simulink model "TP"  (R2021a)
settings: Solver=VariableStepAuto  StartTime=0.0  StopTime=T  MaxStep=0.01  RelTol=1e-6
undefined symbols (not defined in the file): A, A0, A0_, algorithmSelect, b, C, e1, e2, gamma, theta
settings Model: Creator=X-X  LastModifiedBy=fussybaby
settings SolverCC: AlgebraicLoopSolver=TrustRegion
settings DebuggingCC: SFMachineParentedDataDiag=warning

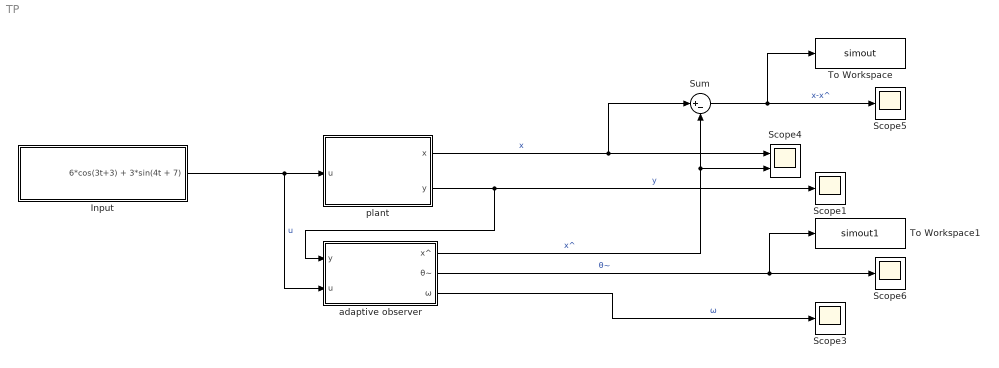
== system TP ==
  Input : Subsystem
  Scope{1,3,5..6} (4 alike) : Scope
  Scope4 : Scope  NumInputPorts=2
  Sum : Sum  Inputs=|+-
  To Workspace : ToWorkspace  VariableName=simout  SaveFormat=Timeseries  SampleTime=-1
  To Workspace1 : ToWorkspace  VariableName=simout1  SaveFormat=Timeseries  SampleTime=-1
  adaptive observer : Subsystem
  plant : Subsystem
  wires:
  plant/2(y) -> Scope1/1, adaptive observer/1(y)  "y"
  Input/1(6*cos(3t+3) + 3*sin(4t + 7)) -> plant/1(u), adaptive observer/2(u)  "u"
  plant/1(x) -> Scope4/1, Sum/1  "x"
  adaptive observer/1(x^) -> Scope4/2, Sum/2  "x^"
  adaptive observer/2(θ~) -> To Workspace1/1, Scope6/1  "θ~"
  adaptive observer/3(ω) -> Scope3/1  "ω"
  Sum/1 -> To Workspace/1, Scope5/1  "x-x^"

== system TP/Input ==
  Sine Wave : Sin  Amplitude=-6  Frequency=3  Phase=3-pi/2  SampleTime=0
  Sine Wave1 : Sin  Amplitude=3  Frequency=4  Phase=7  SampleTime=0
  Sum : Sum  Inputs=|++
  6*cos(3t+3) + 3*sin(4t + 7) : Outport
  wires:
  Sine Wave1/1 -> Sum/2  "3*sin(4t + 7)"
  Sum/1 -> 6*cos(3t+3) + 3*sin(4t + 7)/1
  Sine Wave/1 -> Sum/1  "6*cos(3t+3)"

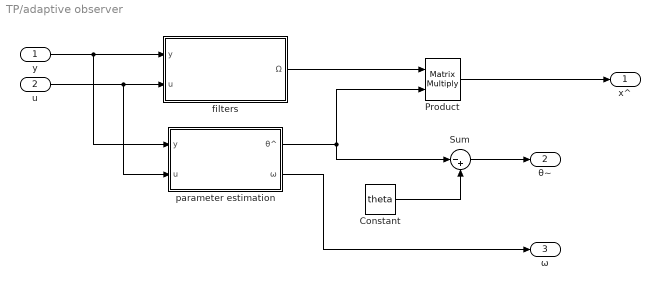
== system TP/adaptive observer ==
  y : Inport
  u : Inport  Port=2
  Constant : Constant  Value=theta
  Product : Product  Multiplication=Matrix(*)
  Sum : Sum  Inputs=|-+
  "filters " : Subsystem
  "parameter estimation " : Subsystem
  x^ : Outport
  θ~ : Outport  Port=2
  ω : Outport  Port=3
  wires:
  Product/1 -> x^/1
  y/1 -> "parameter estimation "/1(y), "filters "/1(y)
  u/1 -> "parameter estimation "/2(u), "filters "/2(u)
  "filters "/1(Ω) -> Product/1
  Constant/1 -> Sum/2
  Sum/1 -> θ~/1
  "parameter estimation "/1(θ^) -> Sum/1, Product/2
  "parameter estimation "/2(ω) -> ω/1

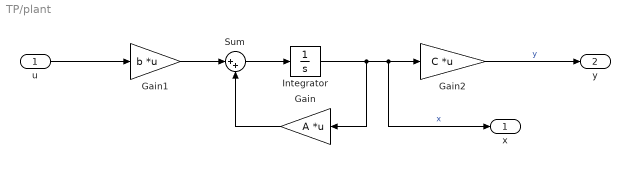
== system TP/plant ==
  u : Inport
  Gain : Gain  Gain=A  Multiplication=Matrix(K*u) (u vector)
  Gain1 : Gain  Gain=b  Multiplication=Matrix(K*u) (u vector)
  Gain2 : Gain  Gain=C  Multiplication=Matrix(K*u) (u vector)
  Integrator : Integrator  InitialCondition=[1; 0]
  Sum : Sum  Inputs=|++
  x : Outport
  y : Outport  Port=2
  wires:
  Integrator/1 -> x/1, Gain2/1, Gain/1  "x"
  Gain1/1 -> Sum/1
  Gain/1 -> Sum/2
  Sum/1 -> Integrator/1
  u/1 -> Gain1/1
  Gain2/1 -> y/1  "y"

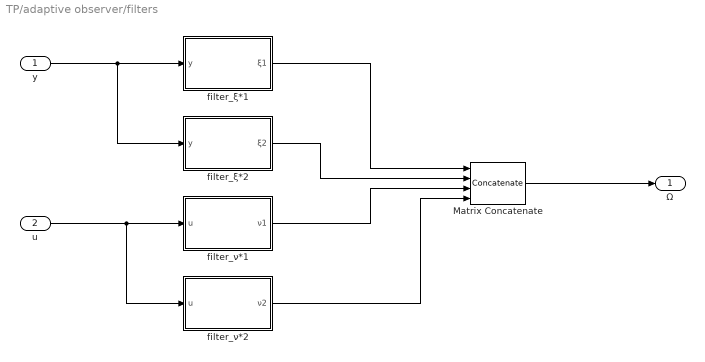
== system TP/adaptive observer/filters  ==
  y : Inport
  u : Inport  Port=2
  Matrix Concatenate : Concatenate  NumInputs=4  Mode=Multidimensional array  ConcatenateDimension=2
  filter_ν*1 : Subsystem
  filter_ν*2 : Subsystem
  filter_ξ*1 : Subsystem
  filter_ξ*2 : Subsystem
  Ω : Outport
  wires:
  y/1 -> filter_ξ*2/1(y), filter_ξ*1/1(y)
  u/1 -> filter_ν*2/1(u), filter_ν*1/1(u)
  filter_ξ*1/1(ξ1) -> Matrix Concatenate/1
  filter_ξ*2/1(ξ2) -> Matrix Concatenate/2
  filter_ν*1/1(ν1) -> Matrix Concatenate/3
  filter_ν*2/1(ν2) -> Matrix Concatenate/4
  Matrix Concatenate/1 -> Ω/1

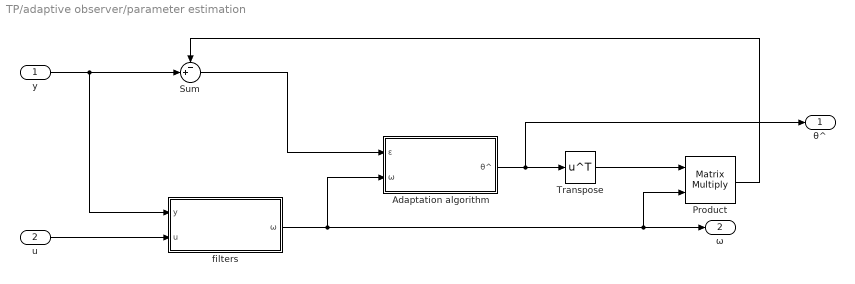
== system TP/adaptive observer/parameter estimation  ==
  y : Inport
  u : Inport  Port=2
  Adaptation algorithm : Subsystem
  Product : Product  Multiplication=Matrix(*)
  Sum : Sum  Inputs=-+|
  Transpose : Math  Operator=transpose  SaturateOnIntegerOverflow=on
  filters : Subsystem
  θ^ : Outport
  ω : Outport  Port=2
  wires:
  u/1 -> filters/2(u)
  filters/1(ω) -> Adaptation algorithm/2(ω), ω/1, Product/2
  Adaptation algorithm/1(θ^) -> θ^/1, Transpose/1
  Transpose/1 -> Product/1
  Product/1 -> Sum/1
  y/1 -> Sum/2, filters/1(y)
  Sum/1 -> Adaptation algorithm/1(ε)

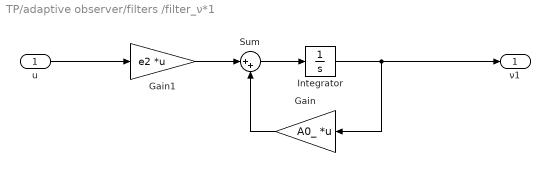
== system TP/adaptive observer/filters /filter_ν*1 ==
  u : Inport
  Gain : Gain  Gain=A0_  Multiplication=Matrix(K*u) (u vector)
  Gain1 : Gain  Gain=e2  Multiplication=Matrix(K*u) (u vector)
  Integrator : Integrator  InitialCondition=[0; 0]
  Sum : Sum  Inputs=|++
  ν1 : Outport
  wires:
  u/1 -> Gain1/1
  Gain/1 -> Sum/2
  Integrator/1 -> ν1/1, Gain/1
  Gain1/1 -> Sum/1
  Sum/1 -> Integrator/1

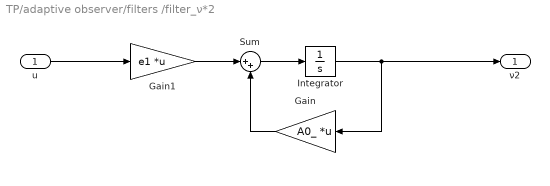
== system TP/adaptive observer/filters /filter_ν*2 ==
  u : Inport
  Gain : Gain  Gain=A0_  Multiplication=Matrix(K*u) (u vector)
  Gain1 : Gain  Gain=e1  Multiplication=Matrix(K*u) (u vector)
  Integrator : Integrator  InitialCondition=[0; 0]
  Sum : Sum  Inputs=|++
  ν2 : Outport
  wires:
  u/1 -> Gain1/1
  Gain/1 -> Sum/2
  Integrator/1 -> ν2/1, Gain/1
  Gain1/1 -> Sum/1
  Sum/1 -> Integrator/1

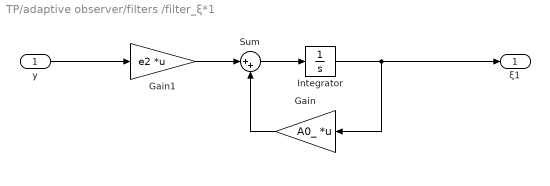
== system TP/adaptive observer/filters /filter_ξ*1 ==
  y : Inport
  Gain : Gain  Gain=A0_  Multiplication=Matrix(K*u) (u vector)
  Gain1 : Gain  Gain=e2  Multiplication=Matrix(K*u) (u vector)
  Integrator : Integrator  InitialCondition=[0; 0]
  Sum : Sum  Inputs=|++
  ξ1 : Outport
  wires:
  y/1 -> Gain1/1
  Gain/1 -> Sum/2
  Integrator/1 -> ξ1/1, Gain/1
  Gain1/1 -> Sum/1
  Sum/1 -> Integrator/1

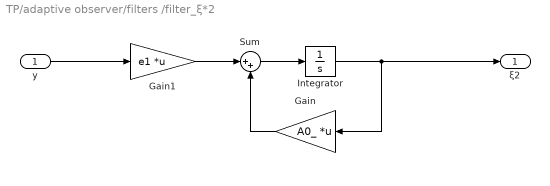
== system TP/adaptive observer/filters /filter_ξ*2 ==
  y : Inport
  Gain : Gain  Gain=A0_  Multiplication=Matrix(K*u) (u vector)
  Gain1 : Gain  Gain=e1  Multiplication=Matrix(K*u) (u vector)
  Integrator : Integrator  InitialCondition=[0; 0]
  Sum : Sum  Inputs=|++
  ξ2 : Outport
  wires:
  y/1 -> Gain1/1
  Gain/1 -> Sum/2
  Integrator/1 -> ξ2/1, Gain/1
  Gain1/1 -> Sum/1
  Sum/1 -> Integrator/1

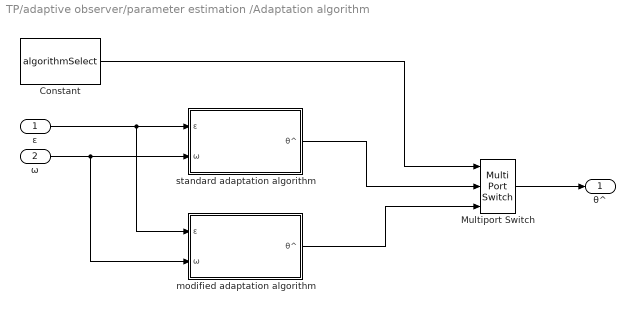
== system TP/adaptive observer/parameter estimation /Adaptation algorithm ==
  ε : Inport
  ω : Inport  Port=2
  Constant : Constant  Value=algorithmSelect
  Multiport Switch : MultiPortSwitch  Inputs=2
  modified adaptation algorithm : Subsystem
  standard adaptation algorithm : Subsystem
  θ^ : Outport
  wires:
  ε/1 -> modified adaptation algorithm/1(ε), standard adaptation algorithm/1(ε)
  ω/1 -> modified adaptation algorithm/2(ω), standard adaptation algorithm/2(ω)
  standard adaptation algorithm/1(θ^) -> Multiport Switch/2
  modified adaptation algorithm/1(θ^) -> Multiport Switch/3
  Constant/1 -> Multiport Switch/1
  Multiport Switch/1 -> θ^/1

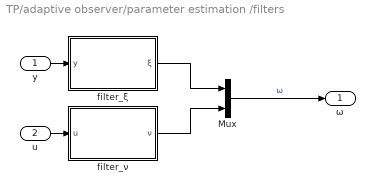
== system TP/adaptive observer/parameter estimation /filters ==
  y : Inport
  u : Inport  Port=2
  Mux : Mux  Inputs=2
  filter_ν : Subsystem
  filter_ξ : Subsystem
  ω : Outport
  wires:
  Mux/1 -> ω/1  "ω"
  filter_ξ/1(ξ) -> Mux/1
  y/1 -> filter_ξ/1(y)
  filter_ν/1(ν) -> Mux/2
  u/1 -> filter_ν/1(u)

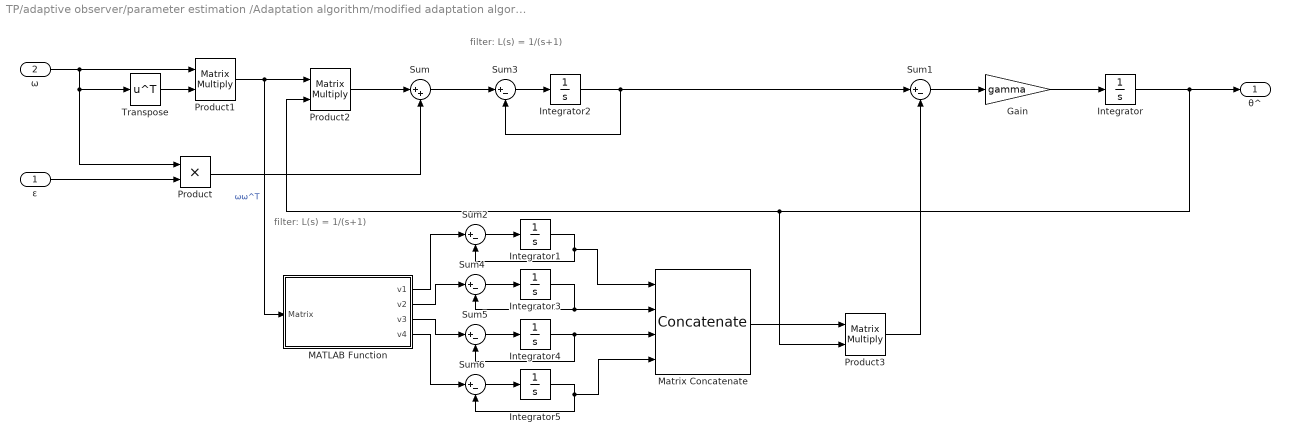
== system TP/adaptive observer/parameter estimation /Adaptation algorithm/modified adaptation algorithm ==
  note: filter: L(s) = 1/(s+1)
  note: filter: L(s) = 1/(s+1)
  ε : Inport
  ω : Inport  Port=2
  Gain : Gain  Gain=gamma
  Integrator{,1..5} (6 alike) : Integrator  InitialCondition=[0; 0; 0; 0]
  MATLAB Function : MATLAB Function  TreatAsAtomicUnit=on
  Matrix Concatenate : Concatenate  NumInputs=4  Mode=Multidimensional array  ConcatenateDimension=2
  Product : Product
  Product1 : Product  Multiplication=Matrix(*)
  Product2 : Product  Multiplication=Matrix(*)
  Product3 : Product  Multiplication=Matrix(*)
  Sum : Sum  Inputs=|++
  Sum{1..6} (6 alike) : Sum  Inputs=|+-
  Transpose : Math  Operator=transpose  SaturateOnIntegerOverflow=on
  θ^ : Outport
  wires:
  Integrator/1 -> Product2/2, Product3/2, θ^/1
  ω/1 -> Product1/1, Transpose/1, Product/1
  Sum1/1 -> Gain/1
  ε/1 -> Product/2
  Gain/1 -> Integrator/1
  Transpose/1 -> Product1/2
  Product1/1 -> MATLAB Function/1(Matrix), Product2/1  "ωω^T"
  Product2/1 -> Sum/1
  Product/1 -> Sum/2
  Product3/1 -> Sum1/2
  Sum3/1 -> Integrator2/1
  Integrator2/1 -> Sum1/1, Sum3/2
  Sum/1 -> Sum3/1
  Sum2/1 -> Integrator1/1
  Integrator1/1 -> Matrix Concatenate/1, Sum2/2
  MATLAB Function/1(v1) -> Sum2/1
  Sum4/1 -> Integrator3/1
  Integrator3/1 -> Sum4/2, Matrix Concatenate/2
  MATLAB Function/2(v2) -> Sum4/1
  Sum5/1 -> Integrator4/1
  Integrator4/1 -> Sum5/2, Matrix Concatenate/3
  MATLAB Function/3(v3) -> Sum5/1
  Sum6/1 -> Integrator5/1
  Integrator5/1 -> Sum6/2, Matrix Concatenate/4
  MATLAB Function/4(v4) -> Sum6/1
  Matrix Concatenate/1 -> Product3/1

== system TP/adaptive observer/parameter estimation /Adaptation algorithm/standard adaptation algorithm ==
  ε : Inport
  ω : Inport  Port=2
  Gain : Gain  Gain=gamma
  Integrator : Integrator  InitialCondition=[0; 0; 0; 0]
  Product : Product
  θ^ : Outport
  wires:
  Integrator/1 -> θ^/1
  Gain/1 -> Integrator/1
  ω/1 -> Product/2
  Product/1 -> Gain/1
  ε/1 -> Product/1

== system TP/adaptive observer/parameter estimation /filters/filter_ν ==
  u : Inport
  Gain : Gain  Gain=A0  Multiplication=Matrix(K*u) (u vector)
  Gain1 : Gain  Gain=e2  Multiplication=Matrix(K*u) (u vector)
  Integrator : Integrator  InitialCondition=[0; 0]
  Sum : Sum  Inputs=|++
  ν : Outport
  wires:
  u/1 -> Gain1/1
  Gain/1 -> Sum/2
  Integrator/1 -> ν/1, Gain/1  "ν"
  Gain1/1 -> Sum/1
  Sum/1 -> Integrator/1

== system TP/adaptive observer/parameter estimation /filters/filter_ξ ==
  y : Inport
  Gain : Gain  Gain=A0  Multiplication=Matrix(K*u) (u vector)
  Gain1 : Gain  Gain=e2  Multiplication=Matrix(K*u) (u vector)
  Integrator : Integrator  InitialCondition=[0; 0]
  Sum : Sum  Inputs=|++
  ξ : Outport
  wires:
  y/1 -> Gain1/1
  Gain/1 -> Sum/2
  Integrator/1 -> ξ/1, Gain/1  "ξ"
  Gain1/1 -> Sum/1
  Sum/1 -> Integrator/1

== matlab function TP/adaptive observer/parameter estimation /Adaptation algorithm/modified adaptation algorithm/MATLAB Function ==
  data: Matrix input; v1 output; v2 output; v3 output; v4 output
function [v1,v2,v3,v4] = matrix2columnVector(Matrix)
v1 = Matrix(:, 1);
v2 = Matrix(:, 2);
v3 = Matrix(:, 3);
v4 = Matrix(:, 4);
end
